simulink subsystem "sub_motores"  (R2023b)
settings: Solver=VariableStepAuto  StartTime=0.0  StopTime=10.0  RelTol=1e-3
libraries: arduinolib x6, simulink x2
settings Model: Creator=Daniel  LastModifiedBy=Usuario_UMA

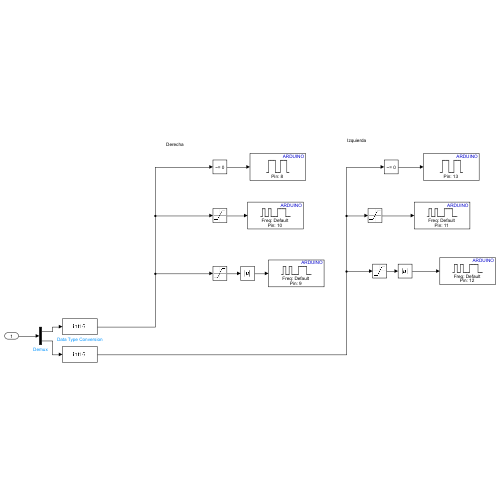
[thumbnail: Simulink's stored preview of the top-level diagram]
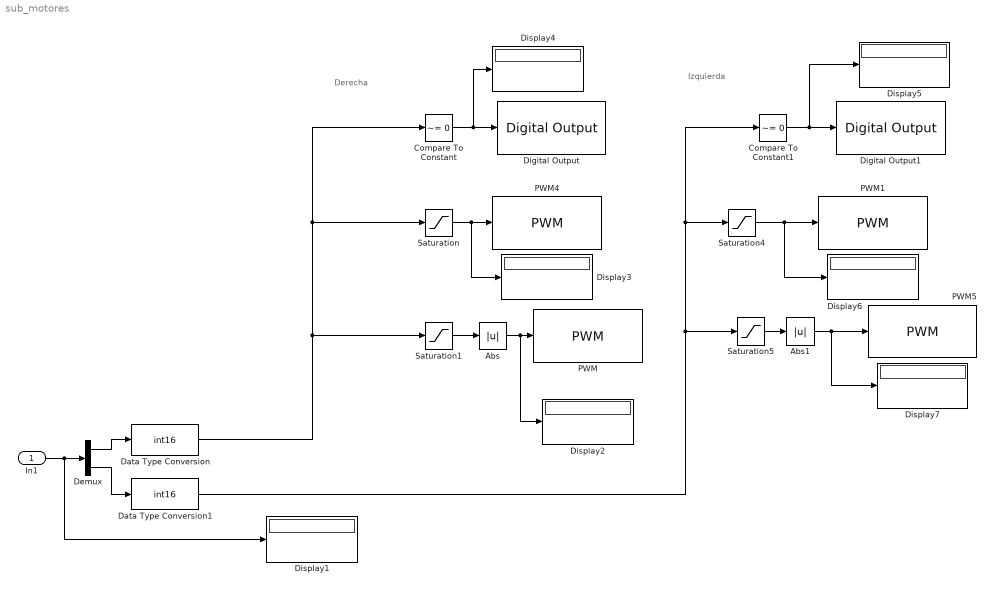
== system sub_motores ==
  note: Izquierda
  note: Derecha
  In1 : Inport
  Abs : Abs  SaturateOnIntegerOverflow=off
  Abs1 : Abs  SaturateOnIntegerOverflow=off
  Compare To Constant : simulink/Logic and Bit Operations/Compare To Constant  relop=~=  const=0  OutDataTypeStr=boolean
  Compare To Constant1 : simulink/Logic and Bit Operations/Compare To Constant  relop=~=  const=0  OutDataTypeStr=boolean
  Data Type Conversion : DataTypeConversion  OutDataTypeStr=int16  SaturateOnIntegerOverflow=off  RndMeth=Floor
  Data Type Conversion1 : DataTypeConversion  OutDataTypeStr=int16  SaturateOnIntegerOverflow=off  RndMeth=Floor
  Demux : Demux  Outputs=2
  Digital Output : arduinolib/Digital Output  pinNumber=8  Direction=output  blockPlatform=arduino
  Digital Output1 : arduinolib/Digital Output  pinNumber=13  Direction=output  blockPlatform=arduino
  Display{1..7} (7 alike) : Display
  PWM : arduinolib/PWM  pinNumber=9  frequencyType=Default  desiredFrequency=490.2  achievableFrequency=490.2
  PWM1 : arduinolib/PWM  pinNumber=11  frequencyType=Default  desiredFrequency=490.2  achievableFrequency=490.2
  PWM4 : arduinolib/PWM  pinNumber=10  frequencyType=Default  desiredFrequency=490.2  achievableFrequency=490.2
  PWM5 : arduinolib/PWM  pinNumber=12  frequencyType=Default  desiredFrequency=490.2  achievableFrequency=490.2
  Saturation : Saturate  UpperLimit=255  LowerLimit=0
  Saturation1 : Saturate  UpperLimit=0  LowerLimit=-255
  Saturation4 : Saturate  UpperLimit=255  LowerLimit=0
  Saturation5 : Saturate  UpperLimit=0  LowerLimit=-255
  wires:
  Compare To Constant1/1 -> Digital Output1/1, Display5/1
  Saturation5/1 -> Abs1/1
  In1/1 -> Demux/1, Display1/1
  Saturation1/1 -> Abs/1
  Compare To Constant/1 -> Digital Output/1, Display4/1
  Abs1/1 -> PWM5/1, Display7/1
  Saturation4/1 -> PWM1/1, Display6/1
  Abs/1 -> PWM/1, Display2/1
  Saturation/1 -> PWM4/1, Display3/1
  Demux/1 -> Data Type Conversion/1
  Demux/2 -> Data Type Conversion1/1
  Data Type Conversion/1 -> Saturation1/1, Saturation/1, Compare To Constant/1
  Data Type Conversion1/1 -> Saturation5/1, Saturation4/1, Compare To Constant1/1
